simulink model "generic_truck"  (R2025a)
settings: Solver=VariableStepAuto  StartTime=0.0  StopTime=600  FixedStep=0.01  MaxStep=0.001  RelTol=1e-3  EnableMultiTasking=on
libraries: TruckMaker4SL x205, simulink x1
(part 5 of 9)

== system generic_truck/TruckMaker/IPG Vehicle/CarAndTrailer/Forces/Suspension Forces/CreateBus Suspension Forces CtrlOut ==
  note: <Your model here>
  In : Inport
  Bus Creator{,1..3,11..14,19..22} (12 alike) : BusCreator  Inputs=4
  Bus Creator9 : BusCreator  Inputs=12
  Demux : Demux  Outputs=12
  Demux{2..5,10..13,18..21} (12 alike) : Demux
  Out : Outport
  wires:
  Demux/3 -> Demux4/1  "RL"
  Demux12/3 -> Bus Creator13/3  "FL2 StabiCtrlOut"
  Demux3/1 -> Bus Creator1/1  "FR SpringCtrlOut"
  Demux3/4 -> Bus Creator1/4  "FR BufferCtrlOut"
  Demux21/2 -> Bus Creator22/2  "RR4 DamperCtrlOut"
  Demux4/3 -> Bus Creator2/3  "RL StabiCtrlOut"
  Demux18/2 -> Bus Creator19/2  "RL3 DamperCtrlOut"
  Demux19/2 -> Bus Creator20/2  "RR3 DamperCtrlOut"
  Demux13/2 -> Bus Creator14/2  "FR2 DamperCtrlOut"
  Demux10/1 -> Bus Creator11/1  "RL2 SpringCtrlOut"
  Demux20/4 -> Bus Creator21/4  "RL4 BufferCtrlOut"
  Demux/5 -> Demux10/1  "RL2"
  Demux20/3 -> Bus Creator21/3  "RL4 StabiCtrlOut"
  Bus Creator1/1 -> Bus Creator9/2
  Bus Creator19/1 -> Bus Creator9/9
  Demux10/3 -> Bus Creator11/3  "RL2 StabiCtrlOut"
  Demux5/1 -> Bus Creator3/1  "RR SpringCtrlOut"
  Demux3/2 -> Bus Creator1/2  "FR DamperCtrlOut"
  Demux13/4 -> Bus Creator14/4  "FR2 BufferCtrlOut"
  Bus Creator2/1 -> Bus Creator9/3
  Demux/12 -> Demux21/1  "RR4"
  Demux/9 -> Demux18/1  "RL3"
  Bus Creator12/1 -> Bus Creator9/6
  Bus Creator20/1 -> Bus Creator9/10
  Demux4/1 -> Bus Creator2/1  "RL SpringCtrlOut"
  Demux12/2 -> Bus Creator13/2  "FL2 DamperCtrlOut"
  Demux12/1 -> Bus Creator13/1  "FL2 SpringCtrlOut"
  Demux/4 -> Demux5/1  "RR"
  Bus Creator13/1 -> Bus Creator9/7
  Demux10/2 -> Bus Creator11/2  "RL2 DamperCtrlOut"
  Bus Creator/1 -> Bus Creator9/1
  Demux18/4 -> Bus Creator19/4  "RL3 BufferCtrlOut"
  Demux11/1 -> Bus Creator12/1  "RR2 SpringCtrlOut"
  Demux2/2 -> Bus Creator/2  "FL DamperCtrlOut"
  Demux13/3 -> Bus Creator14/3  "FR2 StabiCtrlOut"
  Demux2/4 -> Bus Creator/4  "FL BufferCtrlOut"
  Bus Creator14/1 -> Bus Creator9/8
  Demux21/3 -> Bus Creator22/3  "RR4 StabiCtrlOut"
  Demux18/3 -> Bus Creator19/3  "RL3 StabiCtrlOut"
  Demux20/2 -> Bus Creator21/2  "RL4 DamperCtrlOut"
  Demux5/4 -> Bus Creator3/4  "RR BufferCtrlOut"
  Demux/8 -> Demux13/1  "FR2"
  Demux/7 -> Demux12/1  "FL2"
  Demux20/1 -> Bus Creator21/1  "RL4 SpringCtrlOut"
  Demux21/1 -> Bus Creator22/1  "RR4 SpringCtrlOut"
  Demux13/1 -> Bus Creator14/1  "FR2 SpringCtrlOut"
  Demux5/3 -> Bus Creator3/3  "RR StabiCtrlOut"
  Demux19/3 -> Bus Creator20/3  "RR3 StabiCtrlOut"
  Demux4/2 -> Bus Creator2/2  "RL DamperCtrlOut"
  Demux/6 -> Demux11/1  "RR2"
  Demux18/1 -> Bus Creator19/1  "RL3 SpringCtrlOut"
  Demux3/3 -> Bus Creator1/3  "FR StabiCtrlOut"
  Demux/11 -> Demux20/1  "RL4"
  Bus Creator22/1 -> Bus Creator9/12
  Demux10/4 -> Bus Creator11/4  "RL2 BufferCtrlOut"
  Bus Creator11/1 -> Bus Creator9/5
  Bus Creator3/1 -> Bus Creator9/4
  Demux5/2 -> Bus Creator3/2  "RR DamperCtrlOut"
  Bus Creator21/1 -> Bus Creator9/11
  Demux/1 -> Demux2/1  "FL"
  Demux19/4 -> Bus Creator20/4  "RR3 BufferCtrlOut"
  Demux/10 -> Demux19/1  "RR3"
  Demux19/1 -> Bus Creator20/1  "RR3 SpringCtrlOut"
  Demux/2 -> Demux3/1  "FR"
  Demux2/3 -> Bus Creator/3  "FL StabiCtrlOut"
  Demux21/4 -> Bus Creator22/4  "RR4 BufferCtrlOut"
  Demux12/4 -> Bus Creator13/4  "FL2 BufferCtrlOut"
  Demux11/2 -> Bus Creator12/2  "RR2 DamperCtrlOut"
  Demux2/1 -> Bus Creator/1  "FL SpringCtrlOut"
  Demux4/4 -> Bus Creator2/4  "RL BufferCtrlOut"
  Demux11/3 -> Bus Creator12/3  "RR2 StabiCtrlOut"
  Demux11/4 -> Bus Creator12/4  "RR2 BufferCtrlOut"
  In/1 -> Demux/1
  Bus Creator9/1 -> Out/1

== system generic_truck/TruckMaker/IPG Vehicle/CarAndTrailer/Forces/Suspension Forces/Damper CreateBus CtrlOutOpt ==
  note: <Your model here>
  In : Inport
  Bus Creator{,1..3,11..14,19..22} (12 alike) : BusCreator  Inputs=4
  Bus Creator9 : BusCreator  Inputs=12
  Demux : Demux  Outputs=12
  Demux{2..5,10..13,18..21} (12 alike) : Demux
  Out : Outport
  wires:
  Demux/8 -> Demux13/1  "FR2"
  Demux19/1 -> Bus Creator20/1  "RR3 CtrlOutOpt0"
  Demux19/3 -> Bus Creator20/3  "RR3 CtrlOutOpt2"
  Demux18/4 -> Bus Creator19/4  "RL3 CtrlOutOpt3"
  Demux2/3 -> Bus Creator/3  "FL CtrlOutOpt2"
  Demux4/4 -> Bus Creator2/4  "RL CtrlOutOpt3"
  Demux3/2 -> Bus Creator1/2  "FR CtrlOutOpt1"
  Bus Creator11/1 -> Bus Creator9/5
  Demux2/4 -> Bus Creator/4  "FL CtrlOutOpt3"
  Demux/9 -> Demux18/1  "RL3"
  Demux10/3 -> Bus Creator11/3  "RL2 CtrlOutOpt2"
  Demux2/1 -> Bus Creator/1  "FL CtrlOutOpt0"
  Demux13/4 -> Bus Creator14/4  "FR2 CtrlOutOpt3"
  Demux19/4 -> Bus Creator20/4  "RR3 CtrlOutOpt3"
  Bus Creator1/1 -> Bus Creator9/2
  Bus Creator14/1 -> Bus Creator9/8
  Demux4/3 -> Bus Creator2/3  "RL CtrlOutOpt2"
  Demux2/2 -> Bus Creator/2  "FL CtrlOutOpt1"
  Demux5/1 -> Bus Creator3/1  "RR CtrlOutOpt0"
  Demux18/3 -> Bus Creator19/3  "RL3 CtrlOutOpt2"
  Demux12/1 -> Bus Creator13/1  "FL2 CtrlOutOpt0"
  Demux12/3 -> Bus Creator13/3  "FL2 CtrlOutOpt2"
  Bus Creator19/1 -> Bus Creator9/9
  Demux4/1 -> Bus Creator2/1  "RL CtrlOutOpt0"
  Demux10/1 -> Bus Creator11/1  "RL2 CtrlOutOpt0"
  Bus Creator/1 -> Bus Creator9/1
  Demux11/1 -> Bus Creator12/1  "RR2 CtrlOutOpt0"
  Demux20/1 -> Bus Creator21/1  "RL4 CtrlOutOpt0"
  Demux10/4 -> Bus Creator11/4  "RL2 CtrlOutOpt3"
  Bus Creator12/1 -> Bus Creator9/6
  Demux12/2 -> Bus Creator13/2  "FL2 CtrlOutOpt1"
  Demux11/3 -> Bus Creator12/3  "RR2 CtrlOutOpt2"
  Demux3/4 -> Bus Creator1/4  "FR CtrlOutOpt3"
  Demux18/2 -> Bus Creator19/2  "RL3 CtrlOutOpt1"
  Demux5/3 -> Bus Creator3/3  "RR CtrlOutOpt2"
  Demux19/2 -> Bus Creator20/2  "RR3 CtrlOutOpt1"
  Bus Creator20/1 -> Bus Creator9/10
  Demux20/2 -> Bus Creator21/2  "RL4 CtrlOutOpt1"
  Demux/7 -> Demux12/1  "FL2"
  Bus Creator2/1 -> Bus Creator9/3
  Demux/4 -> Demux5/1  "RR"
  Demux/1 -> Demux2/1  "FL"
  Demux20/4 -> Bus Creator21/4  "RL4 CtrlOutOpt3"
  Demux13/1 -> Bus Creator14/1  "FR2 CtrlOutOpt0"
  Demux/3 -> Demux4/1  "RL"
  Demux20/3 -> Bus Creator21/3  "RL4 CtrlOutOpt2"
  Demux3/1 -> Bus Creator1/1  "FR CtrlOutOpt0"
  Demux21/4 -> Bus Creator22/4  "RR4 CtrlOutOpt3"
  Demux11/4 -> Bus Creator12/4  "RR2 CtrlOutOpt3"
  Demux3/3 -> Bus Creator1/3  "FR CtrlOutOpt2"
  Demux18/1 -> Bus Creator19/1  "RL3 CtrlOutOpt0"
  Demux/10 -> Demux19/1  "RR3"
  Demux10/2 -> Bus Creator11/2  "RL2 CtrlOutOpt1"
  Demux12/4 -> Bus Creator13/4  "FL2 CtrlOutOpt3"
  Demux13/3 -> Bus Creator14/3  "FR2 CtrlOutOpt2"
  Demux4/2 -> Bus Creator2/2  "RL CtrlOutOpt1"
  Demux21/2 -> Bus Creator22/2  "RR4 CtrlOutOpt1"
  Demux5/2 -> Bus Creator3/2  "RR CtrlOutOpt1"
  Bus Creator3/1 -> Bus Creator9/4
  Demux21/3 -> Bus Creator22/3  "RR4 CtrlOutOpt2"
  Demux21/1 -> Bus Creator22/1  "RR4 CtrlOutOpt0"
  Demux/6 -> Demux11/1  "RR2"
  Demux/2 -> Demux3/1  "FR"
  Demux11/2 -> Bus Creator12/2  "RR2 CtrlOutOpt1"
  Demux13/2 -> Bus Creator14/2  "FR2 CtrlOutOpt1"
  Demux/5 -> Demux10/1  "RL2"
  Bus Creator13/1 -> Bus Creator9/7
  Demux5/4 -> Bus Creator3/4  "RR CtrlOutOpt3"
  In/1 -> Demux/1
  Bus Creator9/1 -> Out/1
  Demux/11 -> Demux20/1  "RL4"
  Bus Creator21/1 -> Bus Creator9/11
  Demux/12 -> Demux21/1  "RR4"
  Bus Creator22/1 -> Bus Creator9/12

== system generic_truck/TruckMaker/IPG Vehicle/CarAndTrailer/Forces/Suspension Forces/FrcSystem CreateBus CtrlOutOpt ==
  note: <Your model here>
  In : Inport
  Bus Creator9 : BusCreator  Inputs=192
  Demux : Demux  Outputs=192
  Out : Outport
  wires:
  In/1 -> Demux/1
  Bus Creator9/1 -> Out/1
  Demux/64 -> Bus Creator9/64  "CtrlOutOpt63"
  Demux/1 -> Bus Creator9/1  "CtrlOutOpt0"
  Demux/2 -> Bus Creator9/2  "CtrlOutOpt1"
  Demux/3 -> Bus Creator9/3  "CtrlOutOpt2"
  Demux/4 -> Bus Creator9/4  "CtrlOutOpt3"
  Demux/5 -> Bus Creator9/5  "CtrlOutOpt4"
  Demux/6 -> Bus Creator9/6  "CtrlOutOpt5"
  Demux/7 -> Bus Creator9/7  "CtrlOutOpt6"
  Demux/8 -> Bus Creator9/8  "CtrlOutOpt7"
  Demux/9 -> Bus Creator9/9  "CtrlOutOpt8"
  Demux/10 -> Bus Creator9/10  "CtrlOutOpt9"
  Demux/11 -> Bus Creator9/11  "CtrlOutOpt10"
  Demux/12 -> Bus Creator9/12  "CtrlOutOpt11"
  Demux/13 -> Bus Creator9/13  "CtrlOutOpt12"
  Demux/14 -> Bus Creator9/14  "CtrlOutOpt13"
  Demux/15 -> Bus Creator9/15  "CtrlOutOpt14"
  Demux/16 -> Bus Creator9/16  "CtrlOutOpt15"
  Demux/17 -> Bus Creator9/17  "CtrlOutOpt16"
  Demux/18 -> Bus Creator9/18  "CtrlOutOpt17"
  Demux/19 -> Bus Creator9/19  "CtrlOutOpt18"
  Demux/20 -> Bus Creator9/20  "CtrlOutOpt19"
  Demux/21 -> Bus Creator9/21  "CtrlOutOpt20"
  Demux/22 -> Bus Creator9/22  "CtrlOutOpt21"
  Demux/23 -> Bus Creator9/23  "CtrlOutOpt22"
  Demux/24 -> Bus Creator9/24  "CtrlOutOpt23"
  Demux/25 -> Bus Creator9/25  "CtrlOutOpt24"
  Demux/26 -> Bus Creator9/26  "CtrlOutOpt25"
  Demux/27 -> Bus Creator9/27  "CtrlOutOpt26"
  Demux/28 -> Bus Creator9/28  "CtrlOutOpt27"
  Demux/29 -> Bus Creator9/29  "CtrlOutOpt28"
  Demux/30 -> Bus Creator9/30  "CtrlOutOpt29"
  Demux/31 -> Bus Creator9/31  "CtrlOutOpt30"
  Demux/32 -> Bus Creator9/32  "CtrlOutOpt31"
  Demux/33 -> Bus Creator9/33  "CtrlOutOpt32"
  Demux/34 -> Bus Creator9/34  "CtrlOutOpt33"
  Demux/35 -> Bus Creator9/35  "CtrlOutOpt34"
  Demux/36 -> Bus Creator9/36  "CtrlOutOpt35"
  Demux/37 -> Bus Creator9/37  "CtrlOutOpt36"
  Demux/38 -> Bus Creator9/38  "CtrlOutOpt37"
  Demux/39 -> Bus Creator9/39  "CtrlOutOpt38"
  Demux/40 -> Bus Creator9/40  "CtrlOutOpt39"
  Demux/41 -> Bus Creator9/41  "CtrlOutOpt40"
  Demux/42 -> Bus Creator9/42  "CtrlOutOpt41"
  Demux/43 -> Bus Creator9/43  "CtrlOutOpt42"
  Demux/44 -> Bus Creator9/44  "CtrlOutOpt43"
  Demux/45 -> Bus Creator9/45  "CtrlOutOpt44"
  Demux/46 -> Bus Creator9/46  "CtrlOutOpt45"
  Demux/47 -> Bus Creator9/47  "CtrlOutOpt46"
  Demux/48 -> Bus Creator9/48  "CtrlOutOpt47"
  Demux/49 -> Bus Creator9/49  "CtrlOutOpt48"
  Demux/50 -> Bus Creator9/50  "CtrlOutOpt49"
  Demux/51 -> Bus Creator9/51  "CtrlOutOpt50"
  Demux/52 -> Bus Creator9/52  "CtrlOutOpt51"
  Demux/53 -> Bus Creator9/53  "CtrlOutOpt52"
  Demux/54 -> Bus Creator9/54  "CtrlOutOpt53"
  Demux/55 -> Bus Creator9/55  "CtrlOutOpt54"
  Demux/56 -> Bus Creator9/56  "CtrlOutOpt55"
  Demux/57 -> Bus Creator9/57  "CtrlOutOpt56"
  Demux/58 -> Bus Creator9/58  "CtrlOutOpt57"
  Demux/59 -> Bus Creator9/59  "CtrlOutOpt58"
  Demux/60 -> Bus Creator9/60  "CtrlOutOpt59"
  Demux/61 -> Bus Creator9/61  "CtrlOutOpt60"
  Demux/62 -> Bus Creator9/62  "CtrlOutOpt61"
  Demux/63 -> Bus Creator9/63  "CtrlOutOpt62"
  Demux/65 -> Bus Creator9/65  "CtrlOutOpt64"
  Demux/66 -> Bus Creator9/66  "CtrlOutOpt65"
  Demux/67 -> Bus Creator9/67  "CtrlOutOpt66"
  Demux/68 -> Bus Creator9/68  "CtrlOutOpt67"
  Demux/69 -> Bus Creator9/69  "CtrlOutOpt68"
  Demux/70 -> Bus Creator9/70  "CtrlOutOpt69"
  Demux/71 -> Bus Creator9/71  "CtrlOutOpt70"
  Demux/72 -> Bus Creator9/72  "CtrlOutOpt71"
  Demux/73 -> Bus Creator9/73  "CtrlOutOpt72"
  Demux/74 -> Bus Creator9/74  "CtrlOutOpt73"
  Demux/75 -> Bus Creator9/75  "CtrlOutOpt74"
  Demux/76 -> Bus Creator9/76  "CtrlOutOpt75"
  Demux/77 -> Bus Creator9/77  "CtrlOutOpt76"
  Demux/78 -> Bus Creator9/78  "CtrlOutOpt77"
  Demux/79 -> Bus Creator9/79  "CtrlOutOpt78"
  Demux/80 -> Bus Creator9/80  "CtrlOutOpt79"
  Demux/81 -> Bus Creator9/81  "CtrlOutOpt80"
  Demux/82 -> Bus Creator9/82  "CtrlOutOpt81"
  Demux/83 -> Bus Creator9/83  "CtrlOutOpt82"
  Demux/84 -> Bus Creator9/84  "CtrlOutOpt83"
  Demux/85 -> Bus Creator9/85  "CtrlOutOpt84"
  Demux/86 -> Bus Creator9/86  "CtrlOutOpt85"
  Demux/87 -> Bus Creator9/87  "CtrlOutOpt86"
  Demux/88 -> Bus Creator9/88  "CtrlOutOpt87"
  Demux/89 -> Bus Creator9/89  "CtrlOutOpt88"
  Demux/90 -> Bus Creator9/90  "CtrlOutOpt89"
  Demux/91 -> Bus Creator9/91  "CtrlOutOpt90"
  Demux/92 -> Bus Creator9/92  "CtrlOutOpt91"
  Demux/93 -> Bus Creator9/93  "CtrlOutOpt92"
  Demux/94 -> Bus Creator9/94  "CtrlOutOpt93"
  Demux/95 -> Bus Creator9/95  "CtrlOutOpt94"
  Demux/96 -> Bus Creator9/96  "CtrlOutOpt95"
  Demux/97 -> Bus Creator9/97  "CtrlOutOpt96"
  Demux/98 -> Bus Creator9/98  "CtrlOutOpt97"
  Demux/99 -> Bus Creator9/99  "CtrlOutOpt98"
  Demux/100 -> Bus Creator9/100  "CtrlOutOpt99"
  Demux/101 -> Bus Creator9/101  "CtrlOutOpt100"
  Demux/102 -> Bus Creator9/102  "CtrlOutOpt101"
  Demux/103 -> Bus Creator9/103  "CtrlOutOpt102"
  Demux/104 -> Bus Creator9/104  "CtrlOutOpt103"
  Demux/105 -> Bus Creator9/105  "CtrlOutOpt104"
  Demux/106 -> Bus Creator9/106  "CtrlOutOpt105"
  Demux/107 -> Bus Creator9/107  "CtrlOutOpt106"
  Demux/108 -> Bus Creator9/108  "CtrlOutOpt107"
  Demux/109 -> Bus Creator9/109  "CtrlOutOpt108"
  Demux/110 -> Bus Creator9/110  "CtrlOutOpt109"
  Demux/111 -> Bus Creator9/111  "CtrlOutOpt110"
  Demux/112 -> Bus Creator9/112  "CtrlOutOpt111"
  Demux/113 -> Bus Creator9/113  "CtrlOutOpt112"
  Demux/114 -> Bus Creator9/114  "CtrlOutOpt113"
  Demux/115 -> Bus Creator9/115  "CtrlOutOpt114"
  Demux/116 -> Bus Creator9/116  "CtrlOutOpt115"
  Demux/117 -> Bus Creator9/117  "CtrlOutOpt116"
  Demux/118 -> Bus Creator9/118  "CtrlOutOpt117"
  Demux/119 -> Bus Creator9/119  "CtrlOutOpt118"
  Demux/120 -> Bus Creator9/120  "CtrlOutOpt119"
  Demux/121 -> Bus Creator9/121  "CtrlOutOpt120"
  Demux/122 -> Bus Creator9/122  "CtrlOutOpt121"
  Demux/123 -> Bus Creator9/123  "CtrlOutOpt122"
  Demux/124 -> Bus Creator9/124  "CtrlOutOpt123"
  Demux/125 -> Bus Creator9/125  "CtrlOutOpt124"
  Demux/126 -> Bus Creator9/126  "CtrlOutOpt125"
  Demux/127 -> Bus Creator9/127  "CtrlOutOpt126"
  Demux/128 -> Bus Creator9/128  "CtrlOutOpt127"
  Demux/129 -> Bus Creator9/129  "CtrlOutOpt128"
  Demux/130 -> Bus Creator9/130  "CtrlOutOpt129"
  Demux/131 -> Bus Creator9/131  "CtrlOutOpt130"
  Demux/132 -> Bus Creator9/132  "CtrlOutOpt131"
  Demux/133 -> Bus Creator9/133  "CtrlOutOpt132"
  Demux/134 -> Bus Creator9/134  "CtrlOutOpt133"
  Demux/135 -> Bus Creator9/135  "CtrlOutOpt134"
  Demux/136 -> Bus Creator9/136  "CtrlOutOpt135"
  Demux/137 -> Bus Creator9/137  "CtrlOutOpt136"
  Demux/138 -> Bus Creator9/138  "CtrlOutOpt137"
  Demux/139 -> Bus Creator9/139  "CtrlOutOpt138"
  Demux/140 -> Bus Creator9/140  "CtrlOutOpt139"
  Demux/141 -> Bus Creator9/141  "CtrlOutOpt140"
  Demux/142 -> Bus Creator9/142  "CtrlOutOpt141"
  Demux/143 -> Bus Creator9/143  "CtrlOutOpt142"
  Demux/144 -> Bus Creator9/144  "CtrlOutOpt143"
  Demux/145 -> Bus Creator9/145  "CtrlOutOpt144"
  Demux/146 -> Bus Creator9/146  "CtrlOutOpt145"
  Demux/147 -> Bus Creator9/147  "CtrlOutOpt146"
  Demux/148 -> Bus Creator9/148  "CtrlOutOpt147"
  Demux/149 -> Bus Creator9/149  "CtrlOutOpt148"
  Demux/150 -> Bus Creator9/150  "CtrlOutOpt149"
  Demux/151 -> Bus Creator9/151  "CtrlOutOpt150"
  Demux/152 -> Bus Creator9/152  "CtrlOutOpt151"
  Demux/153 -> Bus Creator9/153  "CtrlOutOpt152"
  Demux/154 -> Bus Creator9/154  "CtrlOutOpt153"
  Demux/155 -> Bus Creator9/155  "CtrlOutOpt154"
  Demux/156 -> Bus Creator9/156  "CtrlOutOpt155"
  Demux/157 -> Bus Creator9/157  "CtrlOutOpt156"
  Demux/158 -> Bus Creator9/158  "CtrlOutOpt157"
  Demux/159 -> Bus Creator9/159  "CtrlOutOpt158"
  Demux/160 -> Bus Creator9/160  "CtrlOutOpt159"
  Demux/161 -> Bus Creator9/161  "CtrlOutOpt160"
  Demux/162 -> Bus Creator9/162  "CtrlOutOpt161"
  Demux/163 -> Bus Creator9/163  "CtrlOutOpt162"
  Demux/164 -> Bus Creator9/164  "CtrlOutOpt163"
  Demux/165 -> Bus Creator9/165  "CtrlOutOpt164"
  Demux/166 -> Bus Creator9/166  "CtrlOutOpt165"
  Demux/167 -> Bus Creator9/167  "CtrlOutOpt166"
  Demux/168 -> Bus Creator9/168  "CtrlOutOpt167"
  Demux/169 -> Bus Creator9/169  "CtrlOutOpt168"
  Demux/170 -> Bus Creator9/170  "CtrlOutOpt169"
  Demux/171 -> Bus Creator9/171  "CtrlOutOpt170"
  Demux/172 -> Bus Creator9/172  "CtrlOutOpt171"
  Demux/173 -> Bus Creator9/173  "CtrlOutOpt172"
  Demux/174 -> Bus Creator9/174  "CtrlOutOpt173"
  Demux/175 -> Bus Creator9/175  "CtrlOutOpt174"
  Demux/176 -> Bus Creator9/176  "CtrlOutOpt175"
  Demux/177 -> Bus Creator9/177  "CtrlOutOpt176"
  Demux/178 -> Bus Creator9/178  "CtrlOutOpt177"
  Demux/179 -> Bus Creator9/179  "CtrlOutOpt178"
  Demux/180 -> Bus Creator9/180  "CtrlOutOpt179"
  Demux/181 -> Bus Creator9/181  "CtrlOutOpt180"
  Demux/182 -> Bus Creator9/182  "CtrlOutOpt181"
  Demux/183 -> Bus Creator9/183  "CtrlOutOpt182"
  Demux/184 -> Bus Creator9/184  "CtrlOutOpt183"
  Demux/185 -> Bus Creator9/185  "CtrlOutOpt184"
  Demux/186 -> Bus Creator9/186  "CtrlOutOpt185"
  Demux/187 -> Bus Creator9/187  "CtrlOutOpt186"
  Demux/188 -> Bus Creator9/188  "CtrlOutOpt187"
  Demux/189 -> Bus Creator9/189  "CtrlOutOpt188"
  Demux/190 -> Bus Creator9/190  "CtrlOutOpt189"
  Demux/191 -> Bus Creator9/191  "CtrlOutOpt190"
  Demux/192 -> Bus Creator9/192  "CtrlOutOpt191"

== system generic_truck/TruckMaker/IPG Vehicle/CarAndTrailer/Forces/Suspension Forces/Spring CreateBus CtrlOutOpt ==
  note: <Your model here>
  In : Inport
  Bus Creator{,1..3,11..14,19..22} (12 alike) : BusCreator  Inputs=4
  Bus Creator9 : BusCreator  Inputs=12
  Demux : Demux  Outputs=12
  Demux{2..5,10..13,18..21} (12 alike) : Demux
  Out : Outport
  wires:
  Demux/8 -> Demux13/1  "FR2"
  Demux19/1 -> Bus Creator20/1  "RR3 CtrlOutOpt0"
  Demux19/3 -> Bus Creator20/3  "RR3 CtrlOutOpt2"
  Demux18/4 -> Bus Creator19/4  "RL3 CtrlOutOpt3"
  Demux2/3 -> Bus Creator/3  "FL CtrlOutOpt2"
  Demux4/4 -> Bus Creator2/4  "RL CtrlOutOpt3"
  Demux3/2 -> Bus Creator1/2  "FR CtrlOutOpt1"
  Bus Creator11/1 -> Bus Creator9/5
  Demux2/4 -> Bus Creator/4  "FL CtrlOutOpt3"
  Demux/9 -> Demux18/1  "RL3"
  Demux10/3 -> Bus Creator11/3  "RL2 CtrlOutOpt2"
  Demux2/1 -> Bus Creator/1  "FL CtrlOutOpt0"
  Demux13/4 -> Bus Creator14/4  "FR2 CtrlOutOpt3"
  Demux19/4 -> Bus Creator20/4  "RR3 CtrlOutOpt3"
  Bus Creator1/1 -> Bus Creator9/2
  Bus Creator14/1 -> Bus Creator9/8
  Demux4/3 -> Bus Creator2/3  "RL CtrlOutOpt2"
  Demux2/2 -> Bus Creator/2  "FL CtrlOutOpt1"
  Demux5/1 -> Bus Creator3/1  "RR CtrlOutOpt0"
  Demux18/3 -> Bus Creator19/3  "RL3 CtrlOutOpt2"
  Demux12/1 -> Bus Creator13/1  "FL2 CtrlOutOpt0"
  Demux12/3 -> Bus Creator13/3  "FL2 CtrlOutOpt2"
  Bus Creator19/1 -> Bus Creator9/9
  Demux4/1 -> Bus Creator2/1  "RL CtrlOutOpt0"
  Demux10/1 -> Bus Creator11/1  "RL2 CtrlOutOpt0"
  Bus Creator/1 -> Bus Creator9/1
  Demux11/1 -> Bus Creator12/1  "RR2 CtrlOutOpt0"
  Demux20/1 -> Bus Creator21/1  "RL4 CtrlOutOpt0"
  Demux10/4 -> Bus Creator11/4  "RL2 CtrlOutOpt3"
  Bus Creator12/1 -> Bus Creator9/6
  Demux12/2 -> Bus Creator13/2  "FL2 CtrlOutOpt1"
  Demux11/3 -> Bus Creator12/3  "RR2 CtrlOutOpt2"
  Demux3/4 -> Bus Creator1/4  "FR CtrlOutOpt3"
  Demux18/2 -> Bus Creator19/2  "RL3 CtrlOutOpt1"
  Demux5/3 -> Bus Creator3/3  "RR CtrlOutOpt2"
  Demux19/2 -> Bus Creator20/2  "RR3 CtrlOutOpt1"
  Bus Creator20/1 -> Bus Creator9/10
  Demux20/2 -> Bus Creator21/2  "RL4 CtrlOutOpt1"
  Demux/7 -> Demux12/1  "FL2"
  Bus Creator2/1 -> Bus Creator9/3
  Demux/4 -> Demux5/1  "RR"
  Demux/1 -> Demux2/1  "FL"
  Demux20/4 -> Bus Creator21/4  "RL4 CtrlOutOpt3"
  Demux13/1 -> Bus Creator14/1  "FR2 CtrlOutOpt0"
  Demux/3 -> Demux4/1  "RL"
  Demux20/3 -> Bus Creator21/3  "RL4 CtrlOutOpt2"
  Demux3/1 -> Bus Creator1/1  "FR CtrlOutOpt0"
  Demux21/4 -> Bus Creator22/4  "RR4 CtrlOutOpt3"
  Demux11/4 -> Bus Creator12/4  "RR2 CtrlOutOpt3"
  Demux3/3 -> Bus Creator1/3  "FR CtrlOutOpt2"
  Demux18/1 -> Bus Creator19/1  "RL3 CtrlOutOpt0"
  Demux/10 -> Demux19/1  "RR3"
  Demux10/2 -> Bus Creator11/2  "RL2 CtrlOutOpt1"
  Demux12/4 -> Bus Creator13/4  "FL2 CtrlOutOpt3"
  Demux13/3 -> Bus Creator14/3  "FR2 CtrlOutOpt2"
  Demux4/2 -> Bus Creator2/2  "RL CtrlOutOpt1"
  Demux21/2 -> Bus Creator22/2  "RR4 CtrlOutOpt1"
  Demux5/2 -> Bus Creator3/2  "RR CtrlOutOpt1"
  Bus Creator3/1 -> Bus Creator9/4
  Demux21/3 -> Bus Creator22/3  "RR4 CtrlOutOpt2"
  Demux21/1 -> Bus Creator22/1  "RR4 CtrlOutOpt0"
  Demux/6 -> Demux11/1  "RR2"
  Demux/2 -> Demux3/1  "FR"
  Demux11/2 -> Bus Creator12/2  "RR2 CtrlOutOpt1"
  Demux13/2 -> Bus Creator14/2  "FR2 CtrlOutOpt1"
  Demux/5 -> Demux10/1  "RL2"
  Bus Creator13/1 -> Bus Creator9/7
  Demux5/4 -> Bus Creator3/4  "RR CtrlOutOpt3"
  In/1 -> Demux/1
  Bus Creator9/1 -> Out/1
  Demux/11 -> Demux20/1  "RL4"
  Bus Creator21/1 -> Bus Creator9/11
  Demux/12 -> Demux21/1  "RR4"
  Bus Creator22/1 -> Bus Creator9/12

== system generic_truck/TruckMaker/IPG Vehicle/CarAndTrailer/Forces/Suspension Forces/Stabi CreateBus CtrlOutOpt ==
  note: <Your model here>
  In : Inport
  Bus Creator{,1..3,11..14,19..22} (12 alike) : BusCreator  Inputs=4
  Bus Creator9 : BusCreator  Inputs=12
  Demux : Demux  Outputs=12
  Demux{2..5,10..13,18..21} (12 alike) : Demux
  Out : Outport
  wires:
  Demux/8 -> Demux13/1  "FR2"
  Demux19/1 -> Bus Creator20/1  "RR3 CtrlOutOpt0"
  Demux19/3 -> Bus Creator20/3  "RR3 CtrlOutOpt2"
  Demux18/4 -> Bus Creator19/4  "RL3 CtrlOutOpt3"
  Demux2/3 -> Bus Creator/3  "FL CtrlOutOpt2"
  Demux4/4 -> Bus Creator2/4  "RL CtrlOutOpt3"
  Demux3/2 -> Bus Creator1/2  "FR CtrlOutOpt1"
  Bus Creator11/1 -> Bus Creator9/5
  Demux2/4 -> Bus Creator/4  "FL CtrlOutOpt3"
  Demux/9 -> Demux18/1  "RL3"
  Demux10/3 -> Bus Creator11/3  "RL2 CtrlOutOpt2"
  Demux2/1 -> Bus Creator/1  "FL CtrlOutOpt0"
  Demux13/4 -> Bus Creator14/4  "FR2 CtrlOutOpt3"
  Demux19/4 -> Bus Creator20/4  "RR3 CtrlOutOpt3"
  Bus Creator1/1 -> Bus Creator9/2
  Bus Creator14/1 -> Bus Creator9/8
  Demux4/3 -> Bus Creator2/3  "RL CtrlOutOpt2"
  Demux2/2 -> Bus Creator/2  "FL CtrlOutOpt1"
  Demux5/1 -> Bus Creator3/1  "RR CtrlOutOpt0"
  Demux18/3 -> Bus Creator19/3  "RL3 CtrlOutOpt2"
  Demux12/1 -> Bus Creator13/1  "FL2 CtrlOutOpt0"
  Demux12/3 -> Bus Creator13/3  "FL2 CtrlOutOpt2"
  Bus Creator19/1 -> Bus Creator9/9
  Demux4/1 -> Bus Creator2/1  "RL CtrlOutOpt0"
  Demux10/1 -> Bus Creator11/1  "RL2 CtrlOutOpt0"
  Bus Creator/1 -> Bus Creator9/1
  Demux11/1 -> Bus Creator12/1  "RR2 CtrlOutOpt0"
  Demux20/1 -> Bus Creator21/1  "RL4 CtrlOutOpt0"
  Demux10/4 -> Bus Creator11/4  "RL2 CtrlOutOpt3"
  Bus Creator12/1 -> Bus Creator9/6
  Demux12/2 -> Bus Creator13/2  "FL2 CtrlOutOpt1"
  Demux11/3 -> Bus Creator12/3  "RR2 CtrlOutOpt2"
  Demux3/4 -> Bus Creator1/4  "FR CtrlOutOpt3"
  Demux18/2 -> Bus Creator19/2  "RL3 CtrlOutOpt1"
  Demux5/3 -> Bus Creator3/3  "RR CtrlOutOpt2"
  Demux19/2 -> Bus Creator20/2  "RR3 CtrlOutOpt1"
  Bus Creator20/1 -> Bus Creator9/10
  Demux20/2 -> Bus Creator21/2  "RL4 CtrlOutOpt1"
  Demux/7 -> Demux12/1  "FL2"
  Bus Creator2/1 -> Bus Creator9/3
  Demux/4 -> Demux5/1  "RR"
  Demux/1 -> Demux2/1  "FL"
  Demux20/4 -> Bus Creator21/4  "RL4 CtrlOutOpt3"
  Demux13/1 -> Bus Creator14/1  "FR2 CtrlOutOpt0"
  Demux/3 -> Demux4/1  "RL"
  Demux20/3 -> Bus Creator21/3  "RL4 CtrlOutOpt2"
  Demux3/1 -> Bus Creator1/1  "FR CtrlOutOpt0"
  Demux21/4 -> Bus Creator22/4  "RR4 CtrlOutOpt3"
  Demux11/4 -> Bus Creator12/4  "RR2 CtrlOutOpt3"
  Demux3/3 -> Bus Creator1/3  "FR CtrlOutOpt2"
  Demux18/1 -> Bus Creator19/1  "RL3 CtrlOutOpt0"
  Demux/10 -> Demux19/1  "RR3"
  Demux10/2 -> Bus Creator11/2  "RL2 CtrlOutOpt1"
  Demux12/4 -> Bus Creator13/4  "FL2 CtrlOutOpt3"
  Demux13/3 -> Bus Creator14/3  "FR2 CtrlOutOpt2"
  Demux4/2 -> Bus Creator2/2  "RL CtrlOutOpt1"
  Demux21/2 -> Bus Creator22/2  "RR4 CtrlOutOpt1"
  Demux5/2 -> Bus Creator3/2  "RR CtrlOutOpt1"
  Bus Creator3/1 -> Bus Creator9/4
  Demux21/3 -> Bus Creator22/3  "RR4 CtrlOutOpt2"
  Demux21/1 -> Bus Creator22/1  "RR4 CtrlOutOpt0"
  Demux/6 -> Demux11/1  "RR2"
  Demux/2 -> Demux3/1  "FR"
  Demux11/2 -> Bus Creator12/2  "RR2 CtrlOutOpt1"
  Demux13/2 -> Bus Creator14/2  "FR2 CtrlOutOpt1"
  Demux/5 -> Demux10/1  "RL2"
  Bus Creator13/1 -> Bus Creator9/7
  Demux5/4 -> Bus Creator3/4  "RR CtrlOutOpt3"
  In/1 -> Demux/1
  Bus Creator9/1 -> Out/1
  Demux/11 -> Demux20/1  "RL4"
  Bus Creator21/1 -> Bus Creator9/11
  Demux/12 -> Demux21/1  "RR4"
  Bus Creator22/1 -> Bus Creator9/12

== matlab function generic_truck/TruckMaker/Two_TRack_Model/EKF_ONE_TRACK ==
  data: z input; u input; xhat output; Q input; R input; Ts input; P output; Fyf output; Fyr output
function [xhat, P,Fyf,Fyr] = EKF_Bicycle_Full_NoBias(z, u, Q, R, Ts)
% EKF for One-Track / Bicycle Model (No IMU Bias)
% States: x = [vx; vy; r; Cf; Cr]
% Measurements: z = [ax; ay; vx; vy; r; wL; wR]

%% ---------------- Persistent safe initialization ----------------
persistent x Pk initialized

% Säker initialisering
if isempty(x)
    x = [15; 0; 0.05; 2e4; 2e4];  % vx, vy, r, Cf, Cr
end

if isempty(Pk)
    Pk = diag([1 1 0.05 4e4 4e4].^2); % 5x5
end

if isempty(initialized)
    initialized = true;
end


%% ---------------- Vehicle parameters ----------------


%% ---------------- Inputs ----------------
delta = u(1); % steering angle
Fx    = u(2)/Rw;    % longitudinal force

% PARAMETERS
m  = 6800;        %  mass
g  = 9.82;        % gravity contanst   
Jz = 12994.917;   % yaw interia
Rw = 0.49;          % wheel radius
width = 2.49;       % track width

p_cog  = [3.473; 0; 0.925];
p_fax  = [4.520; 0; 0.490];

p_rax  = [0.950; 0; 0.490];
p_imu  = [3.600; 0; 1.000];

lf = abs(p_fax(1)-p_cog(1));   % front CoG distance
lr = abs(p_cog(1)-p_rax(1));   % rear CoG distance
L  = lf + lr;
h  = p_cog(3);

Rfax = p_fax - p_imu; Rfax(3) = -p_imu(3);
Rrax = p_rax - p_imu; Rrax(3) = -p_imu(3);
Rcog = p_cog - p_imu;


% INPUTS
delta = u(1);                             % Average steering Angle (FL +FR)/2
T_rl  = u(2);                             % torque RL  
T_rr  = u(3);                             %torque RR
Rwheel = 0.49;                            % wheel radius
Fx_vehicle = (T_rl + T_rr)/Rwheel;        % longitudinal force

%% ---------------- States ----------------
vx = x(1); vy = x(2); r = x(3); Cf = x(4); Cr= x(5);

Rotf = [ cos(delta)     -sin(delta)     0;
         sin(delta)      cos(delta)     0;
             0              0           1];

v_cog = [vx; vy; 0];
omega = [0;0;r];

% Contact patch velocities
vf = Rotf.' * (v_cog + cross(omega,Rfax));
vr = v_cog + cross(omega,Rrax);

alpha_f = atan2(vf(2), max(abs(vf(1)),0.1));
alpha_r = atan2(vr(2), max(abs(vr(1)),0.1));

% Longitudinal accel estimate to compute the vertikel forces
dvx_temp = Fx_vehicle/m + vy*r;

% Normal forces
Ffz = m*g*lr/L - m*dvx_temp*h/L;
Frz = m*g*lf/L + m*dvx_temp*h/L;

% Tire forces
Fy_f = Cf * alpha_f * Ffz;
Fy_r = Cr * alpha_r * Frz;

% Full dynamics 
dvx = (Fx_vehicle - Fy_f*sin(delta))/m + vy*r;
dvy = (Fy_f*cos(delta) + Fy_r)/m - vx*r;
dr  = (lf*Fy_f*cos(delta) - lr*Fy_r)/Jz;

% State propagation
xdot = [dvx; dvy; dr; 0; 0];
x_pred = x + Ts*xdot;

%% ---------------- Jacobian F ----------------
F= zeros(5,5);
F(1,:) = [                                1 - (Cf*Ts*sin(delta)*(vy + lf*r))/(m*vx^2),              Ts*(r + (Cf*sin(delta))/(m*vx)),                   Ts*(vy + (Cf*lf*sin(delta))/(m*vx)),    -(Ts*sin(delta)*(delta - (vy + lf*r)/vx))/m,                            0];
F(2,:) = [  -Ts*(r - ((Cr*(vy - lr*r))/vx^2 + (Cf*cos(delta)*(vy + lf*r))/vx^2)/m),      1 - (Ts*(Cr/vx + (Cf*cos(delta))/vx))/m,    -Ts*(vx - ((Cr*lr)/vx - (Cf*lf*cos(delta))/vx)/m),     (Ts*cos(delta)*(delta - (vy + lf*r)/vx))/m,    -(Ts*(vy - lr*r))/(m*vx)];
F(3,:) = [-(Ts*((Cr*lr*(vy - lr*r))/vx^2 - (Cf*lf*cos(delta)*(vy + lf*r))/vx^2))/Jz, (Ts*((Cr*lr)/vx - (Cf*lf*cos(delta))/vx))/Jz, 1 - (Ts*((Cf*cos(delta)*lf^2)/vx + (Cr*lr^2)/vx))/Jz, (Ts*lf*cos(delta)*(delta - (vy + lf*r)/vx))/Jz, (Ts*lr*(vy - lr*r))/(Jz*vx)];
F(4,:) = [                                                                            0,                                              0,                                                      0,                                                 1,                            0];
F(5,:) = [                                                                            0,                                              0,                                                      0,                                                 0,                            1];


%% ---------------- Covariance prediction ----------------
P_pred = F*Pk*F' + Q;

%% ---------------- Measurement model ----------------
ax_hat = dvx -  vy*r;                % longitudinal accel
ay_hat = dvy + vx*r;                % lateral accel
vx_hat = vx;
vy_hat = vy;
r_hat  = r;
wL_hat = (vx - width/2 * r)/Rw;
wR_hat = (vx + width/2 * r)/Rw;

a_cog = [ax_hat; ay_hat; 0];
alpha_vec = [0;0;dr];

% Transform to IMU
a_imu = a_cog - cross(omega, cross(omega,Rcog))- cross(alpha_vec,Rcog);
v_imu = v_cog + cross(omega,Rcog);

z_hat = [a_imu(1:2);
         v_imu(1:2);
         alpha_vec(3);
         omega(3)];

%z_hat = [ax_hat; ay_hat; vx_hat; vy_hat; dr_hat r_hat; wL_hat; wR_hat];

%% ---------------- Measurement Jacobian H ----------------
H = zeros(size(z_hat,1),size(x,1));

%H = zeros(7,5);
H(1,:) = [                               1 - (Cf*Ts*sin(delta)*(vy + lf*r))/(m*vx^2),         Ts*(r + (Cf*sin(delta))/(m*vx)) - r,                      Ts*(vy + (Cf*lf*sin(delta))/(m*vx)) - vy, -(Ts*sin(delta)*(delta - (vy + lf*r)/vx))/m,                            0];
H(2,:) = [-Ts*(r - ((Cr*(vy - lr*r))/vx^2 + (Cf*cos(delta)*(vy + lf*r))/vx^2)/m), 1 - (Ts*(Cr/vx_eff + (Cf*cos(delta))/vx))/m, vx - Ts*(vx - ((Cr*lr)/vx - (Cf*lf*cos(delta))/vx)/m),  (Ts*cos(delta)*(delta - (vy + lf*r)/vx))/m, -(Ts*(vy - lr*r))/(m*vx)];
H(3,:) = [                                                                             1,                                               0,                                                                 0,                                               0,            0];
H(4,:) = [                                                                             0,                                               1,                                                                 0,                                               0,            0];
H(5,:) = [                                                                             0,                                               0,                                                                 0,                                               0,            0];
H(6,:) = [                                                                             0,                                               0,                                                                 1,                                               0,            0];
H(7,:) = [                                                                             1/Rw,                                            0,                                                     -width/(2*Rw),                                               0,            0];
H(8,:) = [                                                                             1/Rw,                                            0,                                                      width/(2*Rw),                                               0,            0];

%% ---------------- EKF update ----------------
S = H*P_pred*H' + R;
K = P_pred*H'/S;

x = x_pred + K*(z - z_hat);
Pk = P_pred - K*S*K';

%% ---------------- Output ----------------
xhat = x;
P = Pk;

end

== matlab function generic_truck/TruckMaker/Two_TRack_Model/MATLAB Function2 ==
  data: z input; u input; vx output; Ts input; vy output; wz output; Cf_est output; Cr_est output; Fyf output; Fyr output
function [vx, vy, wz, Cf_est, Cr_est, Fyf, Fyr] = AdaptiveOneTrackCFCR(z, u, Ts)
% Adaptive one-track model for online estimation of front/rear cornering stiffness
%
% Inputs:
%   z  = [ax; ay; vx; vy; wz] -> sensor measurements
%   u  = [delta; Fx]          -> steering angle (rad), longitudinal force (N)
%   Ts -> sampling time (s)
%
% Outputs:
%   vx, vy, wz      -> vehicle states (m/s, m/s, rad/s)
%   Cf_est, Cr_est  -> estimated front/rear cornering stiffness (N/rad)
%   Fyf, Fyr        -> lateral forces (N)

persistent Cf Cr vx_prev vy_prev wz_prev

%% ---------------- Initialization ----------------
if isempty(vx_prev)
    vx_prev = z(3); vy_prev = z(4); wz_prev = z(5);
end
if isempty(Cf)
    Cf = 15000;  % initial guess
    Cr = 15000;
end

%% ---------------- Vehicle parameters ----------------
m  = 7000;      % mass [kg]
Jz = 14232.357; % yaw inertia [kg*m^2]
lf = 1.12;      % front CoG to axle [m]
lr = 2.45;      % rear CoG to axle [m]
Rw = 0.49;      % wheel radius [m]
track = 2.49;   % track width [m]

%% ---------------- Inputs ----------------
delta = u(1); % steering [rad]
Fx    = u(2); % longitudinal force [N]

%% ---------------- States from sensors ----------------
vx = z(3); 
vy = z(4); 
wz = z(5);

% Protect low velocity
vx_eff = max(abs(vx), 1);

%% ---------------- Slip angles ----------------
alpha_f = (vy + lf*wz)/vx_eff - delta;
alpha_r = (vy - lr*wz)/vx_eff;

%% ---------------- Lateral forces ----------------
Fyf = -Cf * alpha_f;
Fyr = -Cr * alpha_r;

%% ---------------- Approximate derivatives ----------------
% simple backward difference
dv_y = (vy - vy_prev)/Ts;
dw_z = (wz - wz_prev)/Ts;

%% ---------------- Regression for Cf/Cr ----------------
% Linear regression: y = Phi * [Cf; Cr]
y   = [m*(dv_y + vx*wz); Jz*dw_z];
Phi = [alpha_f, alpha_r; lf*alpha_f, -lr*alpha_r];

% Adaptive gain
gamma = 1e3;

theta = [Cf; Cr] + gamma * Phi' * (y - Phi*[Cf; Cr]) * Ts;

% Limit to physical range
Cf = theta(1);%max(min(theta(1), 1e5), 5000);
Cr = theta(2);%max(min(theta(2), 1e5), 5000);

Cf_est = Cf;
Cr_est = Cr;

%% ---------------- Recompute lateral forces ----------------
Fyf = Cf_est * alpha_f;
Fyr = -Cr_est * alpha_r;

%% ---------------- Update previous states ----------------
vx_prev = vx;
vy_prev = vy;
wz_prev = wz;

end

== matlab function generic_truck/TruckMaker/Comparison Block Forces /Comparison Functions  ==
  data: Vec_v input; alpha_f output; Car_w input; delta_f input; Toe_angle input; alpha_r output; CyF input; CyR input; Fy output; Vx_wheel output; Vy_wheel output
function [alpha_f, alpha_r, Fy, Vx_wheel, Vy_wheel] = tire_model_4W_vehicleFrame(Vec_v, Car_w, delta_f,Toe_angle, CyF, CyR)
%TIRE_MODEL_4W_VEHICLEFRAME
%  Beräknar slipvinklar och lateral forces för ett 4-hjuls fordon
%  
%  Input:
%    Vec_v   - [3x1] Vehicle velocity i vehicle frame [Vx; Vy; Vz]
%    Car_w   - [3x1] Vehicle angular rates i vehicle frame [rollRate; pitchRate; yawRate]
%    delta_f - [2x1] Framhjul styrvinklar [delta_FL; delta_FR] (rad)
%    CyF     - [2x1] Framhjul cornering stiffness per wheel
%    CyR     - [2x1] Bakhjul cornering stiffness per wheel
%
%  Output:
%    alpha_f - [2x1] Slipvinkel framhjul [rad]
%    alpha_r - [2x1] Slipvinkel bakhjul [rad]
%    Fy      - [4x1] Lateral force per wheel [N]
%    Vx_wheel, Vy_wheel - [4x1] Hjulhastigheter i hjulens frame

%% ================= PARAMETERS =================
eps_v  = 0.1;   % min velocity för slipvinkel
g = 9.82;       % gravitation [m/s^2]
load_front_axle = 4805.882;   
load_rear_axle  = 2194.118;   

%% ================= GEOMETRY =================
% Kontaktpunkter i vehicle frame
tire_contact_point_FL = [4.52;  1.05; 0]; 
tire_contact_point_FR = [4.52; -1.05; 0];
tire_contact_point_RL = [0.95;  1.05; 0];
tire_contact_point_RR = [0.95; -1.05; 0];

% Reference point (IMU/vehicle CoM)
Vec_coor = [3.6; 0; 1];

% Vektorer från CoM till hjul
rFL = tire_contact_point_FL - Vec_coor;
rFR = tire_contact_point_FR - Vec_coor;
rRL = tire_contact_point_RL - Vec_coor;
rRR = tire_contact_point_RR - Vec_coor;

%% ================= CONTACT PATCH VELOCITY =================
V_FL = Vec_v + cross(Car_w, rFL);
V_FR = Vec_v + cross(Car_w, rFR);
V_RL = Vec_v + cross(Car_w, rRL);
V_RR = Vec_v + cross(Car_w, rRR);

%% ================= TRANSFORM TO WHEEL FRAME =================
% 2D rotation för framhjul
R_FL = [cos(delta_f(1)), sin(delta_f(1));
       -sin(delta_f(1)), cos(delta_f(1))];

R_FR = [cos(delta_f(2)), sin(delta_f(2));
       -sin(delta_f(2)), cos(delta_f(2))];

% Bakhjul (delta=0)
R_RL = eye(2);
R_RR = eye(2);

% Transformera
V_FL_local = R_FL * V_FL(1:2);
V_FR_local = R_FR * V_FR(1:2);
V_RL_local = R_RL * V_RL(1:2);
V_RR_local = R_RR * V_RR(1:2);


Vx_wheel = [V_FL_local(1); V_FR_local(1); V_RL_local(1); V_RR_local(1)];
Vy_wheel = [V_FL_local(2); V_FR_local(2); V_RL_local(2); V_RR_local(2)];

%% ================= SLIP ANGLES =================
Vx_safe = max(abs(Vx_wheel), eps_v);  % förhindrar division med 0
alpha = atan2(Vy_wheel, Vx_safe);

% Fram och bak separering
alpha_f = alpha(1:2); % - Toe_angle(1:2);
alpha_r = alpha(3:4);% + Toe_angle(3:4).*[1;-1];

%% ================= CORNERING STIFFNESS =================
Cy_FL = CyF(1) * load_front_axle * g / 2;
Cy_FR = CyF(2) * load_front_axle * g / 2;

Cy_RL = CyR(1) * load_rear_axle  * g / 2;
Cy_RR = CyR(2) * load_rear_axle  * g / 2;

Cy = [Cy_FL; Cy_FR; Cy_RL; Cy_RR];

%% ================= LATERAL FORCES =================
Fy = -Cy .* alpha;

end

== matlab function generic_truck/TruckMaker/Two_TRack_Model/MATLAB Function3 ==
  data: z input; u input; xhat output; Q input; R input; Ts input; P output; sensor_pos input; F_wheel_pos input; R_wheel_pos input
function [xhat,P] = UKF_5state_4W(z,u,Q,R,Ts,sensor_pos,F_wheel_pos,R_wheel_pos)
% UKF for 4-wheel vehicle
% States: x = [vx; vy; wz; CyF; CyR]
% Measurements: z = [ax; ay; vx; vy; wz; wFL; wFR; wRL; wRR]

persistent x Pk
if isempty(x)
    x = [15; 0; 0.05; 4e4; 4e4]; % initial state
end
if isempty(Pk)
    Pk = diag([1 1 0.01 1e6 1e6]);
end

%% Vehicle parameters
m  = 7000;
Jz = 14232.357;
Rw = 0.49;
g  = 9.82;
track = 2.49;

n = length(x); % state dimension

delta = u(1);      % steering input
Fx_in = u(2)/Rw;   % longitudinal force / wheel radius

%% UKF weights (old style)
W0 = 1 - n/3;
Wi = (1-W0)/(2*n);
gamma = sqrt(n/(1-W0));

%% Sigma points
S = chol(Pk,'lower');
X = zeros(n,2*n+1);
X(:,1) = x;
for i=1:n
    X(:,i+1)   = x + gamma*S(:,i);
    X(:,i+1+n) = x - gamma*S(:,i);
end

%% ------------------- PREDICTION -------------------
X_pred = zeros(n,2*n+1);

for k=1:2*n+1
    vx  = X(1,k);
    vy  = X(2,k);
    wz  = X(3,k);
    CyF = X(4,k);
    CyR = X(5,k);

    Car_v = [vx; vy; 0];
    Car_w = [wx; wy; wz];

    % ---- Wheel velocities at contact patch ----
    V_FL = Car_v + cross(Car_w, F_wheel_pos.FL);
    V_FR = Car_v + cross(Car_w, F_wheel_pos.FR);
    V_RL = Car_v + cross(Car_w, R_wheel_pos.RL);
    V_RR = Car_v + cross(Car_w, R_wheel_pos.RR);

    % ---- Rotate front wheels to wheel frame ----
    R_FL = [ cos(delta)  sin(delta) 0;
            -sin(delta)  cos(delta) 0;
             0           0          1];
    R_FR = R_FL;

    VwfL = R_FL * V_FL;
    VwfR = R_FR * V_FR;

    VwrL = V_RL; % rear wheels no steering
    VwrR = V_RR;

    % ---- Slip angles ----
    alpha_FL = atan2(VwfL(2), VwfL(1));
    alpha_FR = atan2(VwfR(2), VwfR(1));
    alpha_RL = atan2(VwrL(2), VwrL(1));
    alpha_RR = atan2(VwrR(2), VwrR(1));

    % ---- Lateral forces ----
    Fy_FL = -CyF * alpha_FL;
    Fy_FR = -CyF * alpha_FR;
    Fy_RL = -CyR * alpha_RL;
    Fy_RR = -CyR * alpha_RR;

    % Total lateral force & yaw moment
    Fy_total = Fy_FL + Fy_FR + Fy_RL + Fy_RR;
    Mz = F_wheel_pos.FL(1)*Fy_FL + F_wheel_pos.FR(1)*Fy_FR + ...
         R_wheel_pos.RL(1)*Fy_RL + R_wheel_pos.RR(1)*Fy_RR;

    % ---- Dynamics ----
    dvx = Fx_in/m + vy*wz;
    dvy = Fy_total/m - vx*wz;
    dwz = Mz / Jz;

    % Propagate state
    X_pred(:,k) = [vx + Ts*dvx;
                   vy + Ts*dvy;
                   wz + Ts*dwz;
                   CyF;
                   CyR];
end

%% Predicted mean
x_pred = W0*X_pred(:,1);
for k=2:2*n+1
    x_pred = x_pred + Wi*X_pred(:,k);
end

%% Predicted covariance
P_pred = Q;
for k=1:2*n+1
    w = Wi; if k==1, w=W0; end
    dx = X_pred(:,k) - x_pred;
    P_pred = P_pred + w*(dx*dx');
end

%% ------------------- MEASUREMENT -------------------
m_dim = length(z);
Z = zeros(m_dim,2*n+1);

for k=1:2*n+1
    vx  = X_pred(1,k);
    vy  = X_pred(2,k);
    wz  = X_pred(3,k);
    CyF = X_pred(4,k);
    CyR = X_pred(5,k);

    Car_v = [vx; vy; 0];
    Car_w = [0; 0; wz];

    % Velocity at sensor
    V_sensor = Car_v + cross(Car_w, sensor_pos);

    % Acceleration at sensor (approx)
    ax_s = Fx_in/m + vy*wz;
    ay_s = ( -CyF*(atan2(Car_v(2)+wz*F_wheel_pos.FL(2),Car_v(1))) ...
           -CyF*(atan2(Car_v(2)+wz*F_wheel_pos.FR(2),Car_v(1))) ...
           -CyR*(atan2(Car_v(2)+wz*R_wheel_pos.RL(2),Car_v(1))) ...
           -CyR*(atan2(Car_v(2)+wz*R_wheel_pos.RR(2),Car_v(1))) )/m;
    az_s = 0;

    % Wheel speeds
    wFL = V_FL(1)/Rw;
    wFR = V_FR(1)/Rw;
    wRL = V_RL(1)/Rw;
    wRR = V_RR(1)/Rw;

    Z(:,k) = [ax_s; ay_s; vx; vy; wz; wFL; wFR; wRL; wRR];
end

% Predicted measurement mean
z_pred = W0*Z(:,1);
for k=2:2*n+1
    z_pred = z_pred + Wi*Z(:,k);
end

% Measurement covariance & cross-covariance
S_cov = R;
Pxz   = zeros(n,m_dim);
for k=1:2*n+1
    w = Wi; if k==1, w=W0; end
    dz = Z(:,k) - z_pred;
    dx = X_pred(:,k) - x_pred;
    S_cov = S_cov + w*(dz*dz');
    Pxz   = Pxz + w*(dx*dz');
end

% Kalman gain
K = Pxz / (S_cov + 1e-6*eye(m_dim));

% Update
x  = x_pred + K*(z - z_pred);
Pk = P_pred - K*S_cov*K';

xhat = x;
P    = Pk;

end



%%%%%%%%%%%%%%%%%%%%%%%
function [alpha_f, alpha_r, Ffy, Fry, ...
          VfL, VfR, VrL, VrR] = tire_model_4W( ...
          Car_v, Car_w, delta_f, CyF, CyR)

% ------------------------------------------------------------
% INPUTS
% Car_v   = [vx; vy; vz]      (vehicle body frame)
% Car_w   = [0; 0; wz]        (vehicle body frame)
% delta_f = [delta_L; delta_R] (front steering angles)
% CyF     = [Cy_FL; Cy_FR]
% CyR     = [Cy_RL; Cy_RR]
%
% OUTPUTS
% alpha_f = [alpha_FL; alpha_FR]
% alpha_r = [alpha_RL; alpha_RR]
% Ffy     = [Fy_FL; Fy_FR]
% Fry     = [Fy_RL; Fy_RR]
% VwfL etc = velocities in wheel frame
% ------------------------------------------------------------

%% ================= PARAMETERS =================
R = 0.49;                 % wheel radius
g = 9.82;

load_front_axle = 4805.882;
load_rear_axle  = 2194.118;

%% ================= GEOMETRY =================
% Wheel centers in vehicle body frame
tire_coor_Fl = [4.52;  1.05; 0.49];
tire_coor_FR = [4.52; -1.05; 0.49];
tire_coor_Rl = [0.95;  1.05; 0.49];
tire_coor_RR = [0.95; -1.05; 0.49];

Car_coor = [3.6; 0; 1];

% Position vectors CG → wheel center
rFl = tire_coor_Fl - Car_coor;
rFR = tire_coor_FR - Car_coor;
rRl = tire_coor_Rl - Car_coor;
rRR = tire_coor_RR - Car_coor;

% Move to CONTACT PATCH
rFl = rFl + [0;0;-R];
rFR = rFR + [0;0;-R];
rRl = rRl + [0;0;-R];
rRR = rRR + [0;0;-R];

%% ================= VELOCITIES AT CONTACT =================
VfL = Car_v + cross(Car_w, rFl);
VfR = Car_v + cross(Car_w, rFR);
VrL = Car_v + cross(Car_w, rRl);
VrR = Car_v + cross(Car_w, rRR);

%% ================= ROTATE TO WHEEL FRAME =================
% Front left
R_FL = [ cos(delta_f(1))  -sin(delta_f(1)) 0;
        sin(delta_f(1))  cos(delta_f(1)) 0;
         0                0               1];

% Front right
R_FR = [ cos(delta_f(2))  -sin(delta_f(2)) 0;
       sin(delta_f(2))  cos(delta_f(2)) 0;
         0                0               1];

VfL = R_FL * VfL;
VfR = R_FR * VfR;

% Rear wheels (no steering)
%VrL = VrL;
%VrR = VrR;

%% ================= SLIP ANGLES =================
alpha_FL = atan2(VfL(2), VfL(1)); %- delta_f(1);
alpha_FR = atan2(VfR(2), VfR(1));%- delta_f(2);

alpha_RL = atan2(VrL(2), VrL(1));
alpha_RR = atan2(VrR(2), VrR(1));

alpha_f = [alpha_FL; alpha_FR];
alpha_r = [alpha_RL; alpha_RR];

%% ================= CORNERING STIFFNESS =================
Cy_FL = CyF(1) * load_front_axle * g / 2;
Cy_FR = CyF(2) * load_front_axle * g / 2;

Cy_RL = CyR(1) * load_rear_axle * g/2;
Cy_RR = CyR(2) * load_rear_axle * g/2;

%% ================= LATERAL FORCES =================
Fy_FL = -Cy_FL * alpha_FL;
Fy_FR = -Cy_FR * alpha_FR;

Fy_RL = -Cy_RL * alpha_RL;
Fy_RR = -Cy_RR * alpha_RR;

Ffy = [Fy_FL; Fy_FR];
Fry = [Fy_RL; Fy_RR];

end

== matlab function generic_truck/TruckMaker/MATLAB Function1 ==
  data: CarVelocity input; CarOmega input; V_FL output; WheelCamberAngle input
function V_FL = fcn(CarVelocity, CarOmega, WheelCamberAngle)
